simulink model "breakv2"  (R2015a)
settings: Solver=ode3  StartTime=0.0  StopTime=10.0  FixedStep=0.05  RelTol=1e-3
values from neighbouring files (symbols this model uses):
  db = 0.000976    [ABAG.m]
  dg = 0.001953    [ABAG.m]
  eb = 0.75    [ABAG.m]
  eg = 0.5    [ABAG.m]
undefined symbols (not defined in the file or in its folder): alpha, Fw, m, maxtorque, r
settings Model: Creator=s141010  LastModifiedBy=s141010
settings DataIOCC: LimitDataPoints=off

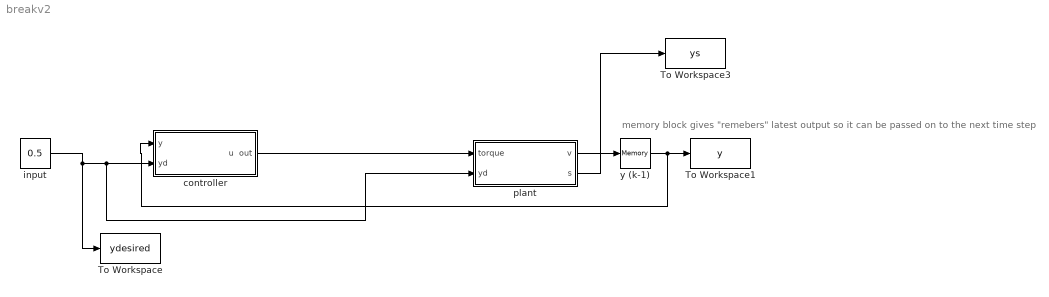
== system breakv2 ==
  note: memory block gives "remebers" latest output so it can be passed on to the next time step
  To Workspace : ToWorkspace  VariableName=ydesired  SaveFormat=Timeseries  SampleTime=-1
  To Workspace1 : ToWorkspace  VariableName=y  SaveFormat=Timeseries  SampleTime=-1
  To Workspace3 : ToWorkspace  VariableName=ys  SaveFormat=Timeseries  SampleTime=-1
  controller : Subsystem
  input : Constant  Value=0.5
  plant : Subsystem
  y (k-1) : Memory
  wires:
  input/1 -> plant/2(yd), controller/2(yd), To Workspace/1
  plant/1(v) -> y (k-1)/1
  y (k-1)/1 -> controller/1(y), To Workspace1/1
  controller/1(u  out) -> plant/1(torque)
  plant/2(s) -> To Workspace3/1

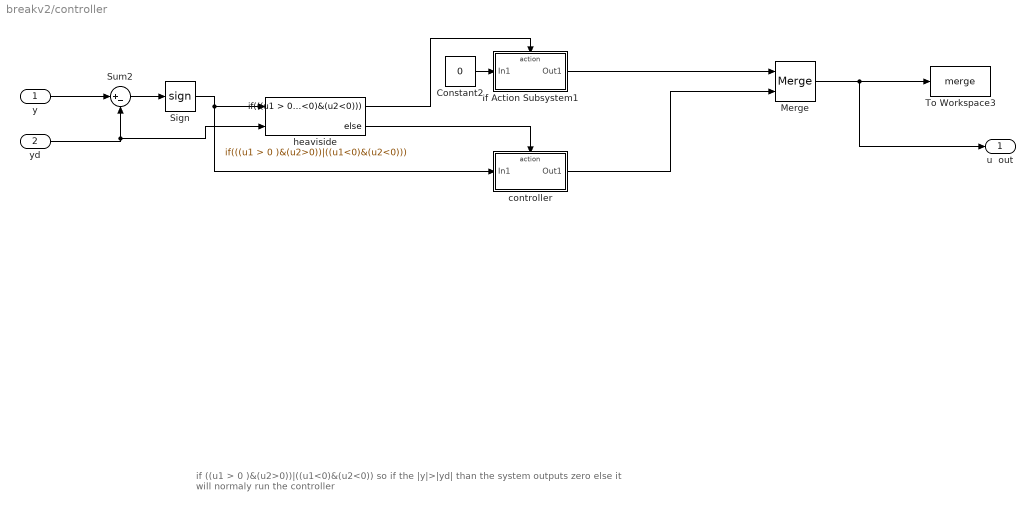
== system breakv2/controller ==
  note: if ((u1 > 0 )&(u2>0))|((u1<0)&(u2<0)) so if the |y|>|yd| than the system outputs zero
      | else it will normaly run the controller
  y : Inport
  yd : Inport  Port=2
  Constant2 : Constant  Value=0
  If Action Subsystem1 : Subsystem  TreatAsAtomicUnit=on
  Merge : Merge
  Sign : Signum
  Sum2 : Sum  Inputs=|+-
  To Workspace3 : ToWorkspace  VariableName=merge  SaveFormat=Timeseries  SampleTime=-1
  controller : Subsystem  TreatAsAtomicUnit=on
  heaviside : If  NumInputs=2  IfExpression=((u1 > 0 )&(u2>0))|((u1<0)&(u2<0))
  u  out : Outport
  wires:
  y/1 -> Sum2/1
  Sum2/1 -> Sign/1
  yd/1 -> heaviside/2, Sum2/2
  Sign/1 -> controller/1(In1), heaviside/1
  Merge/1 -> To Workspace3/1, u  out/1
  Constant2/1 -> If Action Subsystem1/1(In1)
  heaviside/1 -> If Action Subsystem1/Action
  heaviside/2 -> controller/Action
  If Action Subsystem1/1(Out1) -> Merge/1
  controller/1(Out1) -> Merge/2

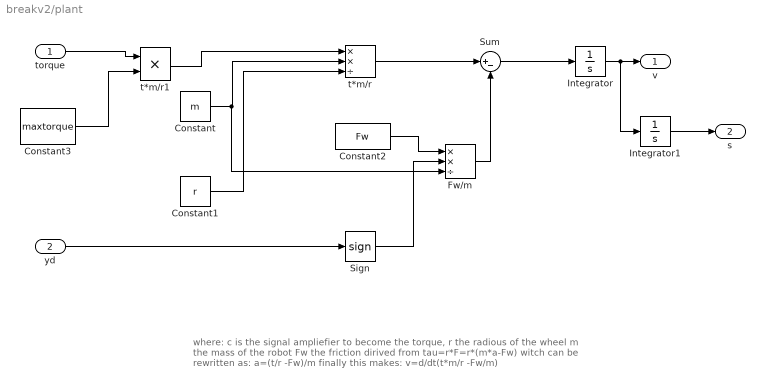
== system breakv2/plant ==
  note: where:
      | c is the signal ampliefier to become the torque,
      | r the radious of the wheel
      | m the mass of the robot
      | Fw the friction
      | dirived from tau=r*F=r*(m*a-Fw)
      | witch can be rewritten as: a=(t/r -Fw)/m
      | finally this makes: v=d/dt(t*m/r -Fw/m)
  torque : Inport
  yd : Inport  Port=2
  Constant : Constant  Value=m
  Constant1 : Constant  Value=r
  Constant2 : Constant  Value=Fw
  Constant3 : Constant  Value=maxtorque
  Fw/m : Product  Inputs=**/
  Integrator : Integrator
  Integrator1 : Integrator
  Sign : Signum  ZeroCross=off
  Sum : Sum  Inputs=|+-
  t*m/r : Product  Inputs=**/
  t*m/r1 : Product  Inputs=**
  v : Outport
  s : Outport  Port=2
  wires:
  Constant/1 -> Fw/m/3, t*m/r/2
  Constant1/1 -> t*m/r/3
  t*m/r/1 -> Sum/1
  Sum/1 -> Integrator/1
  Fw/m/1 -> Sum/2
  Constant2/1 -> Fw/m/1
  Integrator/1 -> Integrator1/1, v/1
  Sign/1 -> Fw/m/2
  yd/1 -> Sign/1
  torque/1 -> t*m/r1/1
  t*m/r1/1 -> t*m/r/1
  Constant3/1 -> t*m/r1/2
  Integrator1/1 -> s/1

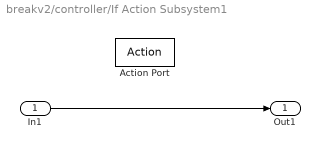
== system breakv2/controller/If Action Subsystem1 ==
  In1 : Inport
  Action Port : ActionPort  ActionType=then
  Out1 : Outport
  wires:
  In1/1 -> Out1/1

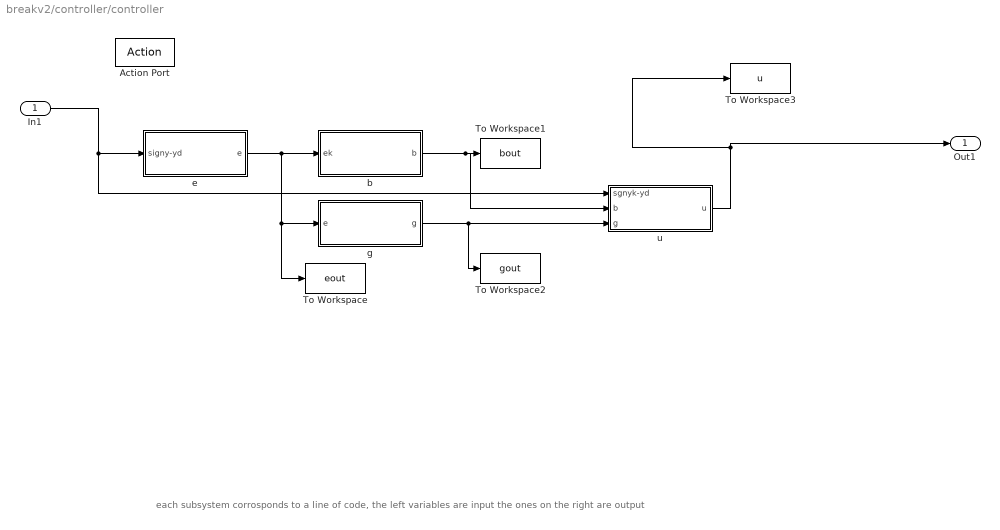
== system breakv2/controller/controller ==
  note: each subsystem corrosponds to a line of code, the left variables are input the ones on the right are output
  In1 : Inport
  Action Port : ActionPort  ActionType=else
  To Workspace : ToWorkspace  VariableName=eout  SaveFormat=Timeseries  SampleTime=-1
  To Workspace1 : ToWorkspace  VariableName=bout  SaveFormat=Timeseries  SampleTime=-1
  To Workspace2 : ToWorkspace  VariableName=gout  SaveFormat=Timeseries  SampleTime=-1
  To Workspace3 : ToWorkspace  VariableName=u  SaveFormat=Timeseries  SampleTime=-1
  b : Subsystem
  e : Subsystem
  g : Subsystem
  u : Subsystem
  Out1 : Outport
  wires:
  e/1(e) -> To Workspace/1, g/1(e), b/1(ek)
  b/1(b) -> u/2(b), To Workspace1/1
  g/1(g) -> To Workspace2/1, u/3(g)
  u/1(u) -> Out1/1, To Workspace3/1
  In1/1 -> u/1(sgnyk-yd), e/1(signy-yd)

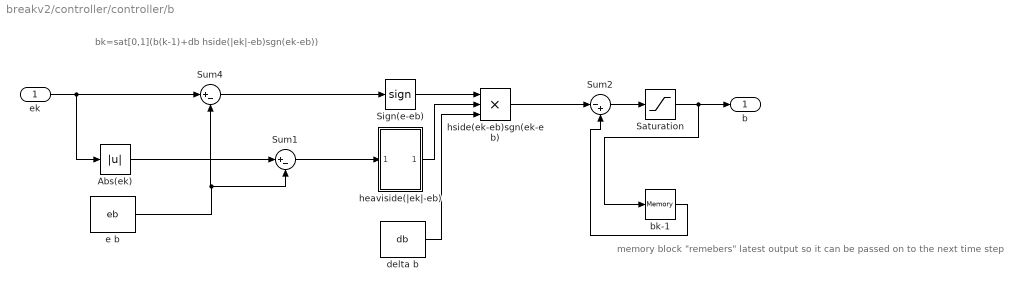
== system breakv2/controller/controller/b ==
  note: bk=sat[0,1](b(k-1)+db hside(|ek|-eb)sgn(ek-eb))
  note: memory block "remebers" latest output so it can be passed on to the next time step
  ek : Inport
  Abs(ek) : Abs
  Saturation : Saturate  UpperLimit=1  LowerLimit=-1
  Sign(e-eb) : Signum  ZeroCross=off
  Sum1 : Sum  Inputs=|+-
  Sum2 : Sum  Inputs=|-+
  Sum4 : Sum  Inputs=|+-
  bk-1 : Memory
  delta b : Constant  Value=db
  e b : Constant  Value=eb
  heaviside(|ek|-eb) : Subsystem
  hside(ek-eb)sgn(ek-eb) : Product  Inputs=3
  b : Outport
  wires:
  ek/1 -> Abs(ek)/1, Sum4/1
  e b/1 -> Sum4/2, Sum1/2
  Sum1/1 -> heaviside(|ek|-eb)/1(In1)
  Abs(ek)/1 -> Sum1/1
  delta b/1 -> hside(ek-eb)sgn(ek-eb)/3
  Sum2/1 -> Saturation/1
  bk-1/1 -> Sum2/2
  Saturation/1 -> bk-1/1, b/1
  heaviside(|ek|-eb)/1(Out1) -> hside(ek-eb)sgn(ek-eb)/2
  hside(ek-eb)sgn(ek-eb)/1 -> Sum2/1
  Sign(e-eb)/1 -> hside(ek-eb)sgn(ek-eb)/1
  Sum4/1 -> Sign(e-eb)/1

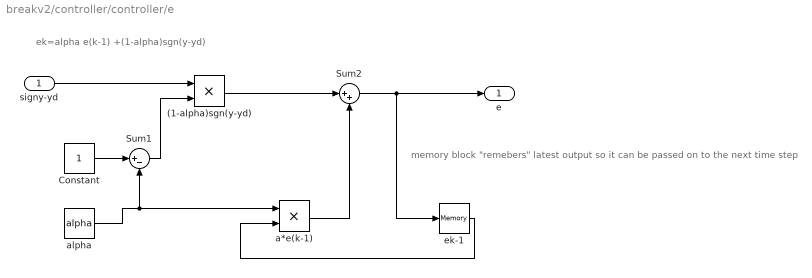
== system breakv2/controller/controller/e ==
  note: ek=alpha e(k-1) +(1-alpha)sgn(y-yd)
  note: memory block "remebers" latest output so it can be passed on to the next time step
  signy-yd : Inport
  (1-alpha)sgn(y-yd) : Product
  Constant : Constant
  Sum1 : Sum  Inputs=|+-
  Sum2 : Sum  Inputs=|++
  a*e(k-1) : Product
  alpha : Constant  Value=alpha
  ek-1 : Memory
  e : Outport
  wires:
  Sum1/1 -> (1-alpha)sgn(y-yd)/2
  Constant/1 -> Sum1/1
  alpha/1 -> a*e(k-1)/1, Sum1/2
  (1-alpha)sgn(y-yd)/1 -> Sum2/1
  signy-yd/1 -> (1-alpha)sgn(y-yd)/1
  a*e(k-1)/1 -> Sum2/2
  Sum2/1 -> ek-1/1, e/1
  ek-1/1 -> a*e(k-1)/2

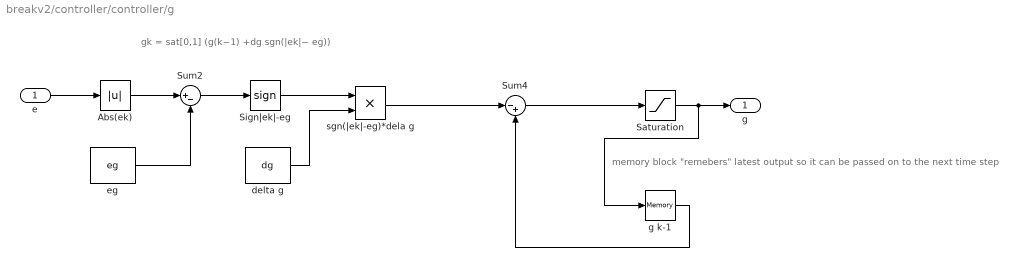
== system breakv2/controller/controller/g ==
  note: gk = sat[0,1] (g(k−1) +dg sgn(|ek|− eg))
  note: memory block "remebers" latest output so it can be passed on to the next time step
  e : Inport
  Abs(ek) : Abs
  Saturation : Saturate  UpperLimit=1  LowerLimit=-1
  Sign|ek|-eg : Signum
  Sum2 : Sum  Inputs=|+-
  Sum4 : Sum  Inputs=|-+
  delta g : Constant  Value=dg
  eg : Constant  Value=eg
  g k-1 : Memory
  sgn(|ek|-eg)*dela g : Product
  g : Outport
  wires:
  e/1 -> Abs(ek)/1
  Saturation/1 -> g k-1/1, g/1
  Abs(ek)/1 -> Sum2/1
  eg/1 -> Sum2/2
  Sign|ek|-eg/1 -> sgn(|ek|-eg)*dela g/1
  delta g/1 -> sgn(|ek|-eg)*dela g/2
  sgn(|ek|-eg)*dela g/1 -> Sum4/1
  Sum4/1 -> Saturation/1
  g k-1/1 -> Sum4/2
  Sum2/1 -> Sign|ek|-eg/1

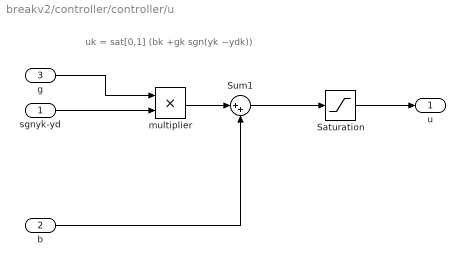
== system breakv2/controller/controller/u ==
  note: uk = sat[0,1] (bk +gk sgn(yk −ydk))
  sgnyk-yd : Inport
  b : Inport  Port=2
  g : Inport  Port=3
  Saturation : Saturate  UpperLimit=1  LowerLimit=-1
  Sum1 : Sum  Inputs=|++
  "multiplier " : Product
  u : Outport
  wires:
  sgnyk-yd/1 -> "multiplier "/2
  "multiplier "/1 -> Sum1/1
  g/1 -> "multiplier "/1
  b/1 -> Sum1/2
  Sum1/1 -> Saturation/1
  Saturation/1 -> u/1

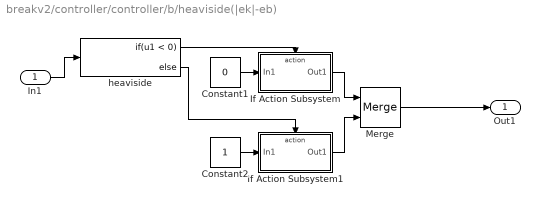
== system breakv2/controller/controller/b/heaviside(|ek|-eb) ==
  In1 : Inport
  Constant1 : Constant  Value=0
  Constant2 : Constant
  If Action Subsystem : Subsystem  TreatAsAtomicUnit=on
  If Action Subsystem1 : Subsystem  TreatAsAtomicUnit=on
  Merge : Merge
  heaviside : If  IfExpression=u1 < 0
  Out1 : Outport
  wires:
  If Action Subsystem1/1(Out1) -> Merge/2
  Constant1/1 -> If Action Subsystem/1(In1)
  Constant2/1 -> If Action Subsystem1/1(In1)
  Merge/1 -> Out1/1
  If Action Subsystem/1(Out1) -> Merge/1
  heaviside/1 -> If Action Subsystem/Action
  heaviside/2 -> If Action Subsystem1/Action
  In1/1 -> heaviside/1

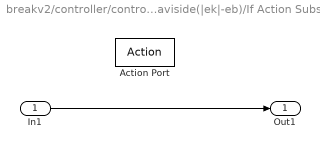
== system breakv2/controller/controller/b/heaviside(|ek|-eb)/If Action Subsystem ==
  In1 : Inport
  Action Port : ActionPort  ActionType=then
  Out1 : Outport
  wires:
  In1/1 -> Out1/1

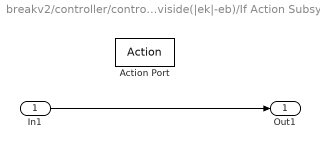
== system breakv2/controller/controller/b/heaviside(|ek|-eb)/If Action Subsystem1 ==
  In1 : Inport
  Action Port : ActionPort  ActionType=else
  Out1 : Outport
  wires:
  In1/1 -> Out1/1
